simulink model "ComparisionOfOpenLoopAndClosedLoopFirstOrderSystemWithGain1"  (R2021a)
settings: Solver=VariableStepAuto  StartTime=0.0  StopTime=10.0  RelTol=1e-3
settings Model: Creator=soumy  LastModifiedBy=soumy

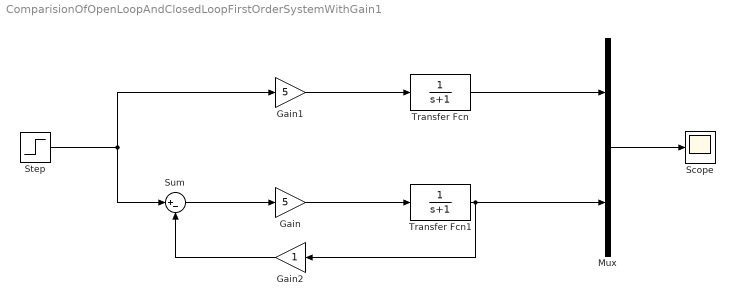
== system ComparisionOfOpenLoopAndClosedLoopFirstOrderSystemWithGain1 ==
  Gain : Gain  Gain=5
  Gain1 : Gain  Gain=5
  Gain2 : Gain
  Mux : Mux  Inputs=2
  Scope : Scope
  Step : Step  SampleTime=0
  Sum : Sum  Inputs=|+-
  Transfer Fcn : TransferFcn  Denominator=[1 1]
  Transfer Fcn1 : TransferFcn  Denominator=[1 1]
  wires:
  Sum/1 -> Gain/1
  Gain/1 -> Transfer Fcn1/1
  Gain1/1 -> Transfer Fcn/1
  Transfer Fcn/1 -> Mux/1
  Transfer Fcn1/1 -> Gain2/1, Mux/2
  Gain2/1 -> Sum/2
  Mux/1 -> Scope/1
  Step/1 -> Sum/1, Gain1/1
